simulink model "drone_udp"  (Simulink 8.4)
settings: Solver=ode45  StartTime=0.0  StopTime=300  FixedStep=.01  RelTol=abstol/10  AbsTol=abstol
undefined symbols (not defined in the file or in its folder): A, Cd, g, I, I_motor, m, MaxPropRate, MaxPwmWidth, MinPwmWidth, q0, r0, r1, r2, r3, r4, RateToForce, rho, v0, w0
libraries: instrumentlib x2, simulink x2, dspmtrx3 x2, aerolibutil x1
settings Model: Creator=Mike  LastModifiedBy=Walker
settings SolverCC: ZeroCrossControl=DisableAll
settings DebuggingCC: StrictBusMsg=Warning

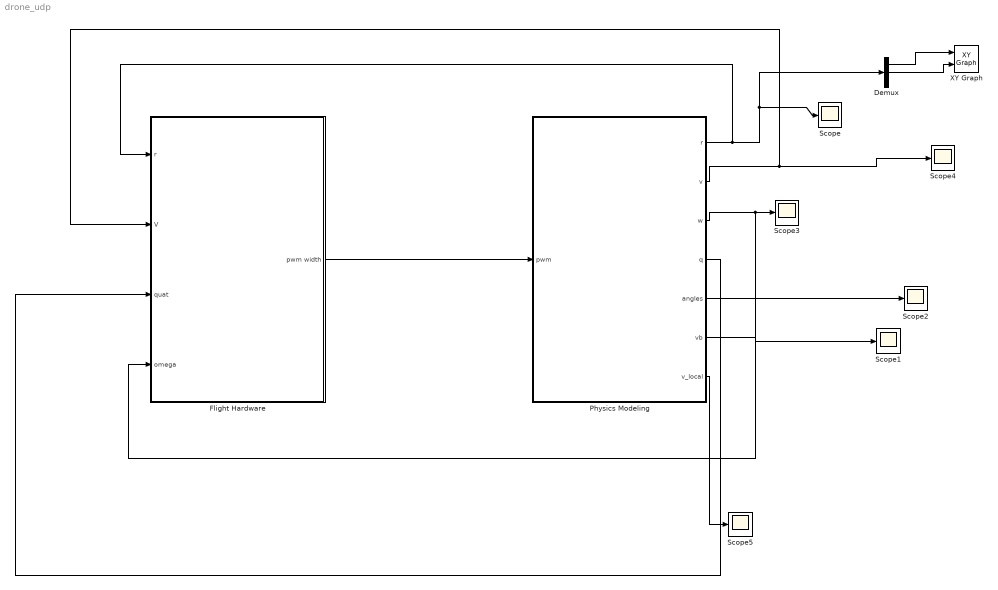
== system drone_udp ==
  Demux : Demux  Outputs=3
  Flight Hardware : Subsystem
  Physics Modeling : Subsystem
  Scope{,1..5} (6 alike) : Scope
      Scope settings: TimeRange=10  YMin=1.25  YMax=5.5
      Scope1 settings: TimeRange=25  YMin=-0.25  YMax=2.75  SaveName=ScopeData7
      Scope2 settings: TimeRange=25  YMin=-0.25  YMax=2.75  SaveName=ScopeData5
      Scope3 settings: TimeRange=50  YMin=-0.0004  YMax=2.5e-005  SaveName=ScopeData13
      Scope4 settings: TimeRange=3.5  YMin=-0.01056459374999874  YMax=0.007040906250001269  SaveName=ScopeData38
      Scope5 settings: TimeRange=25  YMax=65  SaveName=ScopeData10
  XY Graph : simulink/Sinks/XY Graph  xmin=-20  xmax=20  ymin=-20  ymax=20  st=1
  wires:
  Physics Modeling/1(r) -> Scope/1, Demux/1, Flight Hardware/1(r)
  Physics Modeling/5(angles) -> Scope2/1
  Physics Modeling/3(w) -> Scope3/1, Flight Hardware/4(omega)
  Physics Modeling/2(v) -> Scope4/1, Flight Hardware/2(V)
  Physics Modeling/7(v_local) -> Scope5/1
  Physics Modeling/6(vb) -> Scope1/1
  Demux/1 -> XY Graph/1
  Demux/2 -> XY Graph/2
  Flight Hardware/1(pwm width) -> Physics Modeling/1(pwm)
  Physics Modeling/4(q) -> Flight Hardware/3(quat)

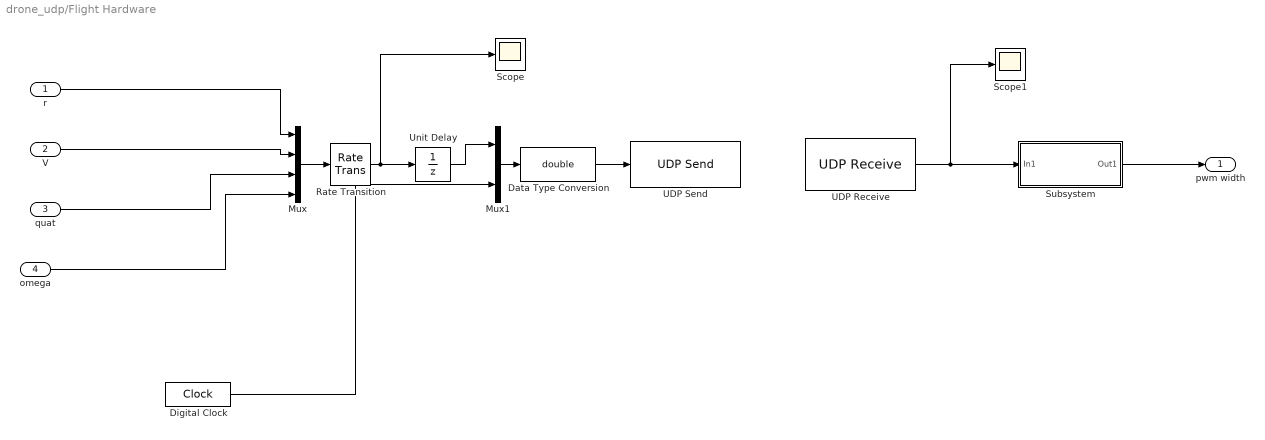
== system drone_udp/Flight Hardware ==
  r : Inport
  V : Inport  Port=2
  quat : Inport  Port=3
  omega : Inport  Port=4
  Data Type Conversion : DataTypeConversion  OutDataTypeStr=double
  Digital Clock : DigitalClock  SampleTime=0.01
  Mux : Mux
  Mux1 : Mux  Inputs=2
  Rate Transition : RateTransition  OutPortSampleTime=0.01
  Scope : Scope
      settings: TimeRange=100
  Scope1 : Scope
      settings: TimeRange=100  YMin=-1e+062  YMax=1e+062  SaveName=ScopeData12
  Subsystem : Subsystem
  UDP Receive : instrumentlib/UDP Receive  Host=127.0.0.1  Port=9091  LocalPort=9091  DataSize=13  EnableBlockingMode=on  Timeout=10  SampleTime=0.01  DataType=double  ByteOrder=LittleEndian
  UDP Send : instrumentlib/UDP Send  Host=127.0.0.1  Port=9090  LocalPort=-1  EnableBlockingMode=off  ByteOrder=LittleEndian
  Unit Delay : UnitDelay  InitialCondition=[r0 v0 q0 w0 ]  SampleTime=-1
  pwm width : Outport
  wires:
  r/1 -> Mux/1
  V/1 -> Mux/2
  omega/1 -> Mux/4
  Data Type Conversion/1 -> UDP Send/1
  quat/1 -> Mux/3
  Mux/1 -> Rate Transition/1
  Rate Transition/1 -> Scope/1, Unit Delay/1
  Subsystem/1(Out1) -> pwm width/1
  UDP Receive/1 -> Scope1/1, Subsystem/1(In1)
  Unit Delay/1 -> Mux1/1
  Digital Clock/1 -> Mux1/2
  Mux1/1 -> Data Type Conversion/1

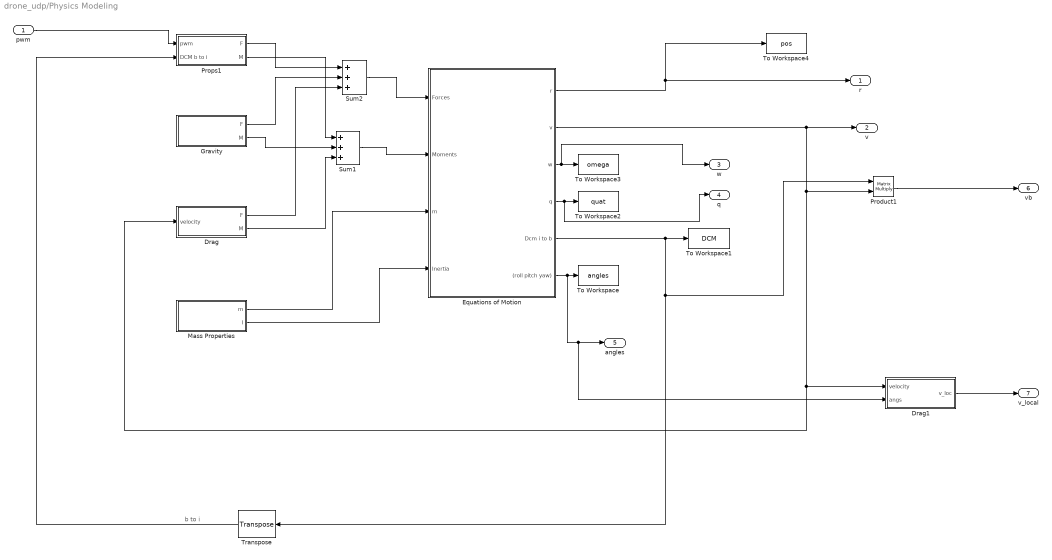
== system drone_udp/Physics Modeling ==
  note: b to i
  pwm : Inport
  Drag : Subsystem
  Drag1 : Subsystem
  Equations of Motion : Subsystem
  Gravity : Subsystem
  Mass Properties : Subsystem
  Product1 : Product  Multiplication=Matrix(*)  RndMeth=Zero
  Props1 : Subsystem
  Sum1 : Sum  Inputs=+++
  Sum2 : Sum  Inputs=+++
  To Workspace : ToWorkspace  VariableName=angles  SampleTime=-1
  To Workspace1 : ToWorkspace  VariableName=DCM  SampleTime=-1
  To Workspace2 : ToWorkspace  VariableName=quat  SampleTime=-1
  To Workspace3 : ToWorkspace  VariableName=omega  SampleTime=-1
  To Workspace4 : ToWorkspace  VariableName=pos  SampleTime=-1
  Transpose : dspmtrx3/Transpose  Hermitian=off  overflowFlag=off
  r : Outport
  v : Outport  Port=2
  w : Outport  Port=3
  q : Outport  Port=4
  angles : Outport  Port=5
  vb : Outport  Port=6
  v_local : Outport  Port=7
  wires:
  Props1/1(F) -> Sum2/1
  Gravity/1(F) -> Sum2/2
  Drag/1(F) -> Sum2/3
  Sum2/1 -> Equations of Motion/1(Forces)
  Props1/2(M) -> Sum1/1
  Gravity/2(M) -> Sum1/2
  Drag/2(M) -> Sum1/3
  Sum1/1 -> Equations of Motion/2(Moments)
  Mass Properties/1(m) -> Equations of Motion/3(m)
  Mass Properties/2(I) -> Equations of Motion/4(Inertia)
  pwm/1 -> Props1/1(pwm)
  Equations of Motion/2(v) -> Drag/1(velocity), Drag1/1(velocity), Product1/2, v/1
  Equations of Motion/1(r) -> To Workspace4/1, r/1
  Equations of Motion/6((roll pitch yaw)) -> To Workspace/1, angles/1, Drag1/2(angs)
  Equations of Motion/5(Dcm i to b) -> To Workspace1/1, Transpose/1, Product1/1
  Equations of Motion/4(q) -> To Workspace2/1, q/1
  Equations of Motion/3(w) -> To Workspace3/1, w/1
  Transpose/1 -> Props1/2("DCM b to i ")
  Product1/1 -> vb/1
  Drag1/1(v_loc) -> v_local/1

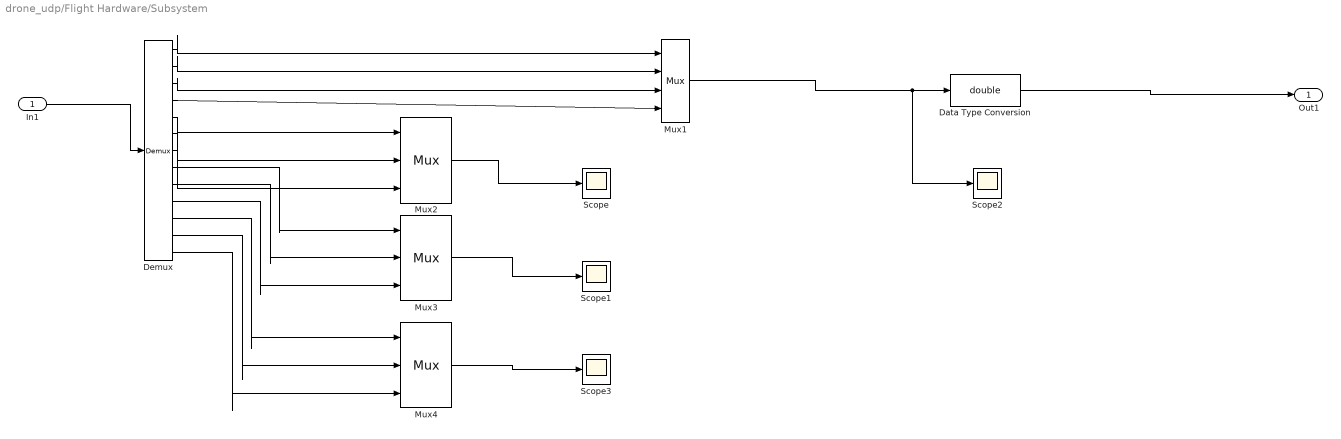
== system drone_udp/Flight Hardware/Subsystem ==
  In1 : Inport
  Data Type Conversion : DataTypeConversion  OutDataTypeStr=double
  Demux : Demux  Outputs=13
  Mux1 : Mux
  Mux2 : Mux  Inputs=3
  Mux3 : Mux  Inputs=3
  Mux4 : Mux  Inputs=3
  Scope{,1..3} (4 alike) : Scope
      Scope settings: YMin=-10  YMax=220  SaveName=ScopeData6
      Scope1 settings: YMin=-1.12743e+008  YMax=-1.02005e+008  SaveName=ScopeData15
      Scope2 settings: TimeRange=3.5  YMin=-2000  YMax=2000  SaveName=ScopeData20
      Scope3 settings: YMin=-0.9  YMax=0.6  SaveName=ScopeData23
  Out1 : Outport
  wires:
  In1/1 -> Demux/1
  Demux/1 -> Mux1/1
  Demux/2 -> Mux1/2
  Demux/3 -> Mux1/3
  Demux/4 -> Mux1/4
  Mux2/1 -> Scope/1
  Demux/5 -> Mux2/1
  Demux/6 -> Mux2/2
  Demux/7 -> Mux2/3
  Data Type Conversion/1 -> Out1/1
  Mux1/1 -> Data Type Conversion/1, Scope2/1
  Demux/8 -> Mux3/1
  Demux/9 -> Mux3/2
  Demux/10 -> Mux3/3
  Mux3/1 -> Scope1/1
  Demux/11 -> Mux4/1
  Demux/12 -> Mux4/2
  Demux/13 -> Mux4/3
  Mux4/1 -> Scope3/1

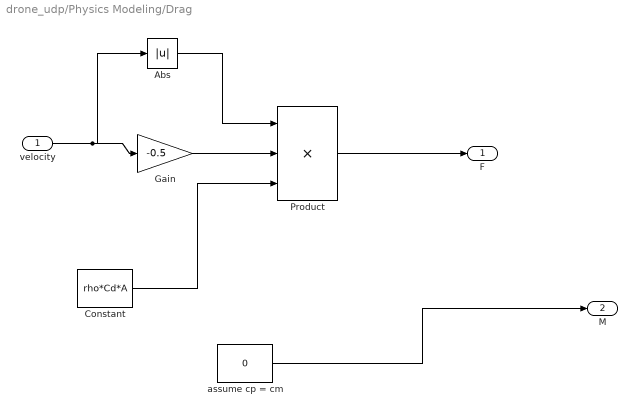
== system drone_udp/Physics Modeling/Drag ==
  velocity : Inport
  Abs : Abs
  Constant : Constant  Value=rho*Cd*A
  Gain : Gain  Gain=-0.5
  Product : Product  Inputs=***  RndMeth=Zero
  assume cp = cm : Constant  Value=0
  F : Outport
  M : Outport  Port=2
  wires:
  velocity/1 -> Abs/1, Gain/1
  Gain/1 -> Product/2
  Abs/1 -> Product/1
  Constant/1 -> Product/3
  assume cp = cm/1 -> M/1
  Product/1 -> F/1

== system drone_udp/Physics Modeling/Drag1 ==
  velocity : Inport
  angs : Inport  Port=2
  Embedded MATLAB Function : MATLAB Function  TreatAsAtomicUnit=on
  Product : Product  Multiplication=Matrix(*)  RndMeth=Zero
  v_loc : Outport
  wires:
  velocity/1 -> Product/2
  Product/1 -> v_loc/1
  angs/1 -> Embedded MATLAB Function/1(u)
  Embedded MATLAB Function/1(y) -> Product/1

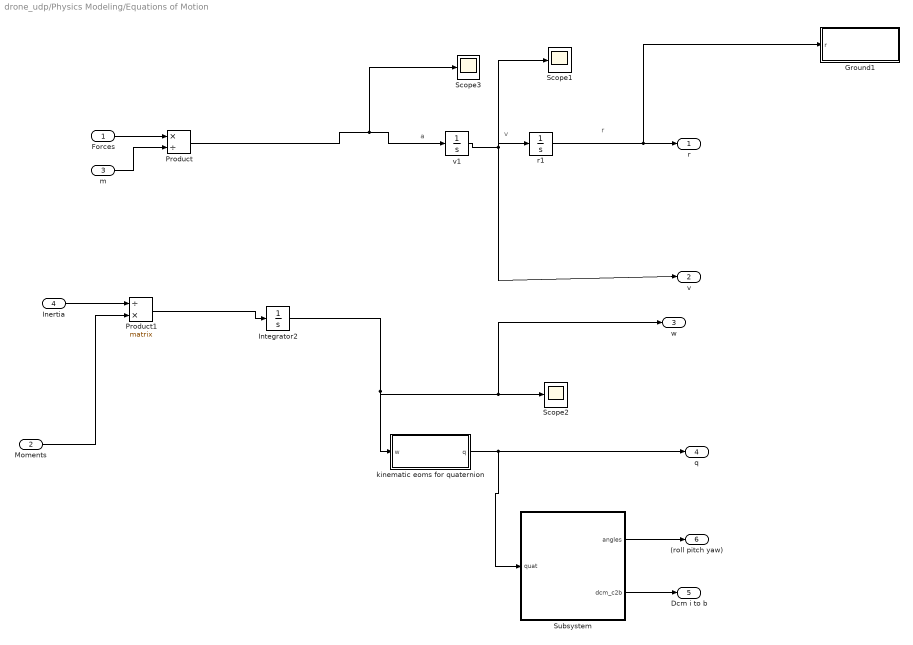
== system drone_udp/Physics Modeling/Equations of Motion ==
  note: a
  note: v
  note: r
  Forces : Inport
  Moments : Inport  Port=2
  m : Inport  Port=3
  Inertia : Inport  Port=4
  Ground1 : Subsystem
  Integrator2 : Integrator  InitialCondition=w0  AbsoluteTolerance=abstol
  Product : Product  Inputs=*/  RndMeth=Zero
  Product1 : Product  Inputs=/*  Multiplication=Matrix(*)  RndMeth=Zero
  Scope1 : Scope
      settings: TimeRange=50  YMin=-2000  YMax=0  SaveName=ScopeData24
  Scope2 : Scope
      settings: TimeRange=50  YMin=-2000  YMax=0  SaveName=ScopeData14
  Scope3 : Scope
      settings: TimeRange=50  YMin=-2000  YMax=0  SaveName=ScopeData25
  Subsystem : Subsystem
  kinematic eoms for quaternion : Subsystem
  r1 : Integrator  InitialCondition=r0  AbsoluteTolerance=abstol
  v1 : Integrator  InitialCondition=v0  AbsoluteTolerance=abstol
  r : Outport
  v : Outport  Port=2
  w : Outport  Port=3
  q : Outport  Port=4
  Dcm i to b : Outport  Port=5
  (roll pitch yaw) : Outport  Port=6
  wires:
  r1/1 -> r/1, Ground1/1(r)
  v1/1 -> r1/1, v/1, Scope1/1
  Forces/1 -> Product/1
  m/1 -> Product/2
  kinematic eoms for quaternion/1(q) -> q/1, Subsystem/1(quat)
  Subsystem/2(dcm_c2b) -> Dcm i to b/1
  Subsystem/1(angles) -> (roll pitch yaw)/1
  Inertia/1 -> Product1/1
  Moments/1 -> Product1/2
  Product/1 -> v1/1, Scope3/1
  Integrator2/1 -> kinematic eoms for quaternion/1(w), Scope2/1, w/1
  Product1/1 -> Integrator2/1

== system drone_udp/Physics Modeling/Gravity ==
  cg=cm in this problem : Constant  Value=0
  mg : Constant  Value=[0;0; -m*g ]
  F : Outport
  M : Outport  Port=2
  wires:
  cg=cm in this problem/1 -> M/1
  mg/1 -> F/1

== system drone_udp/Physics Modeling/Mass Properties ==
  Constant : Constant  Value=m
  a : Constant  Value=I
  m : Outport
  I : Outport  Port=2
  wires:
  a/1 -> I/1
  Constant/1 -> m/1

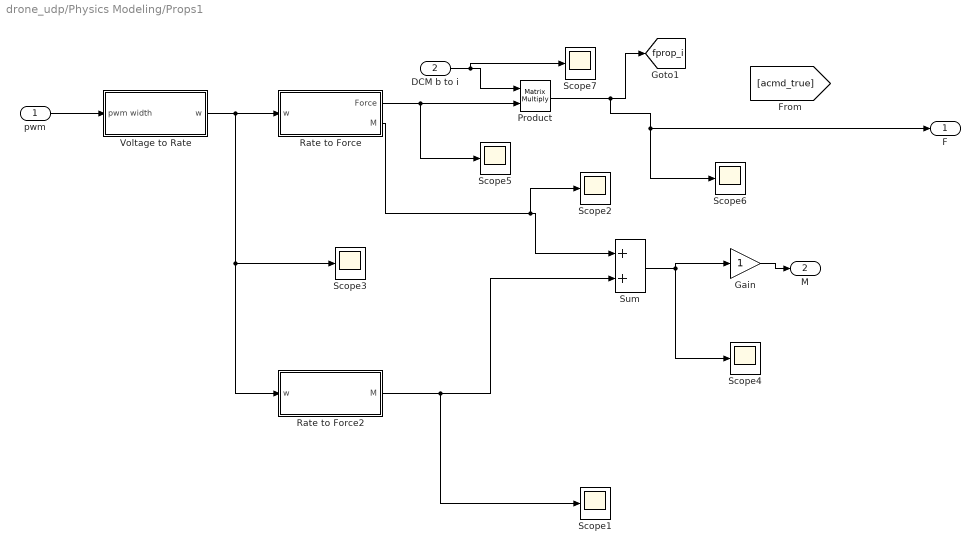
== system drone_udp/Physics Modeling/Props1 ==
  pwm : Inport
  "DCM b to i " : Inport  Port=2
  Gain : Gain
  Product : Product  Multiplication=Matrix(*)  OutDataTypeStr=Inherit: Inherit via back propagation  RndMeth=Nearest
  Rate to Force : Subsystem
  Rate to Force2 : Subsystem
  Scope{1..7} (7 alike) : Scope
      Scope1 settings: TimeRange=50  YMin=0  YMax=200  SaveName=ScopeData2
      Scope2 settings: YMin=-1  YMax=1  SaveName=ScopeData3
      Scope3 settings: TimeRange=50  YMin=2.32987  YMax=2.57513  SaveName=ScopeData4
      Scope4 settings: TimeRange=6.110074626865668  YMin=-3.63961038961039e-009  YMax=-3.405844155844153e-009  SaveName=ScopeData11
      Scope5 settings: TimeRange=50  YMin=0  YMax=40  SaveName=ScopeData9
      Scope6 settings: TimeRange=50  YMin=0  YMax=40  SaveName=ScopeData59
      Scope7 settings: TimeRange=0.2158273381295004  YMin=-0.1758241758241754  YMax=0.1318681318681321  SaveName=ScopeData62
  Sum : Sum
  Voltage to Rate : Subsystem
  F : Outport
  M : Outport  Port=2
  tag scope: fprop_i=global
  wires:
  pwm/1 -> Voltage to Rate/1(pwm width)
  Voltage to Rate/1(w) -> Rate to Force/1(w), Rate to Force2/1(w), Scope3/1
  Sum/1 -> Scope4/1, Gain/1
  Rate to Force/2(M) -> Sum/1, Scope2/1
  Rate to Force2/1(M) -> Sum/2, Scope1/1
  Product/1 -> [fprop_i], Scope6/1, F/1
  "DCM b to i "/1 -> Product/1, Scope7/1
  Rate to Force/1(Force) -> Product/2, Scope5/1
  Gain/1 -> M/1

== system drone_udp/Physics Modeling/Equations of Motion/Ground1 ==
  r : Inport
  Compare To Zero : simulink/Logic and Bit Operations/Compare To Zero  SystemSampleTime=-1  relop=<=  LogicOutDataTypeMode=boolean  ZeroCross=off
  Demux : Demux  Outputs=3
  Stop Simulation : Stop
  Terminator : Terminator
  Terminator1 : Terminator
  wires:
  r/1 -> Demux/1
  Demux/1 -> Terminator/1
  Demux/2 -> Terminator1/1
  Demux/3 -> Compare To Zero/1
  Compare To Zero/1 -> Stop Simulation/1

== system drone_udp/Physics Modeling/Equations of Motion/Subsystem ==
  note: Based on Prof Howell AAE 440 Notes
  note: C is row notation so transpose it!
  quat : Inport
  Transpose1 : dspmtrx3/Transpose  SystemSampleTime=-1  Hermitian=off  overflowFlag=off
  solve direction cosine matrix : Subsystem
  angles : Outport
  dcm_c2b : Outport  Port=2
  wires:
  quat/1 -> solve direction cosine matrix/1(quat)
  solve direction cosine matrix/2(roll pitch yaw) -> angles/1
  solve direction cosine matrix/1(C) -> Transpose1/1
  Transpose1/1 -> dcm_c2b/1

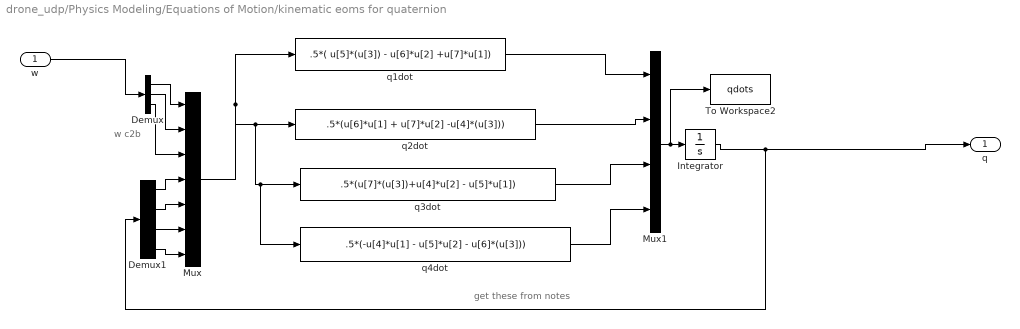
== system drone_udp/Physics Modeling/Equations of Motion/kinematic eoms for quaternion ==
  note: get these from notes
  note: w c2b
  w : Inport
  Demux : Demux  Outputs=3
  Demux1 : Demux
  Integrator : Integrator  InitialCondition=q0  IgnoreLimit=on
  Mux : Mux  Inputs=7
  Mux1 : Mux
  To Workspace2 : ToWorkspace  VariableName=qdots  SampleTime=-1
  q1dot : Fcn  Expr=.5*( u[5]*(u[3]) - u[6]*u[2] +u[7]*u[1])
  q2dot : Fcn  Expr=.5*(u[6]*u[1] + u[7]*u[2] -u[4]*(u[3]))
  q3dot : Fcn  Expr=.5*(u[7]*(u[3])+u[4]*u[2] - u[5]*u[1])
  q4dot : Fcn  Expr=.5*(-u[4]*u[1] - u[5]*u[2] - u[6]*(u[3]))
  q : Outport
  wires:
  Mux1/1 -> Integrator/1, To Workspace2/1
  Integrator/1 -> Demux1/1, q/1
  q4dot/1 -> Mux1/4
  q3dot/1 -> Mux1/3
  q2dot/1 -> Mux1/2
  q1dot/1 -> Mux1/1
  Mux/1 -> q1dot/1, q2dot/1, q3dot/1, q4dot/1
  w/1 -> Demux/1
  Demux/1 -> Mux/1
  Demux/2 -> Mux/2
  Demux/3 -> Mux/3
  Demux1/1 -> Mux/4
  Demux1/2 -> Mux/5
  Demux1/3 -> Mux/6
  Demux1/4 -> Mux/7

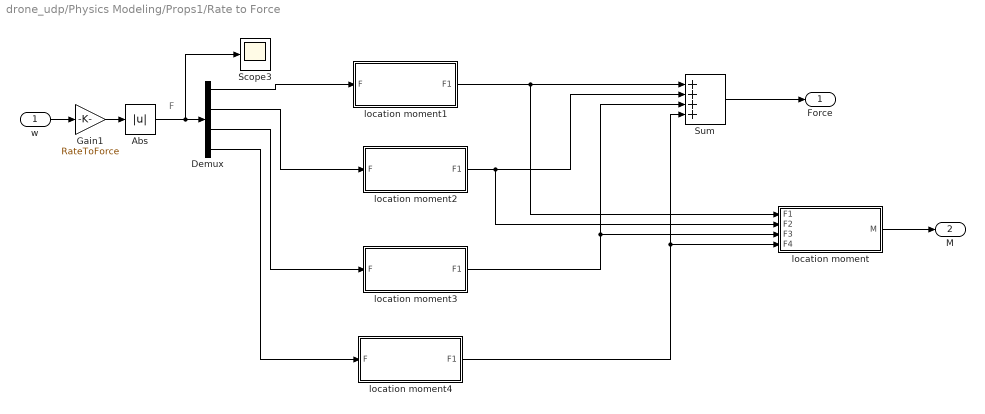
== system drone_udp/Physics Modeling/Props1/Rate to Force ==
  note: F
  w : Inport
  Abs : Abs
  Demux : Demux
  Gain1 : Gain  Gain=RateToForce
  Scope3 : Scope
      settings: TimeRange=50  YMin=2.32987  YMax=2.57513  SaveName=ScopeData8
  Sum : Sum  Inputs=++++
  location moment : Subsystem
  location moment1 : Subsystem
  location moment2 : Subsystem
  location moment3 : Subsystem
  location moment4 : Subsystem
  Force : Outport
  M : Outport  Port=2
  wires:
  location moment/1(M) -> M/1
  Sum/1 -> Force/1
  location moment1/1(F1) -> Sum/1, location moment/1(F1)
  location moment2/1(F1) -> Sum/2, location moment/2(F2)
  location moment3/1(F1) -> Sum/3, location moment/3(F3)
  location moment4/1(F1) -> Sum/4, location moment/4(F4)
  Demux/1 -> location moment1/1(F)
  Demux/2 -> location moment2/1(F)
  Demux/3 -> location moment3/1(F)
  Demux/4 -> location moment4/1(F)
  Abs/1 -> Demux/1, Scope3/1
  w/1 -> Gain1/1
  Gain1/1 -> Abs/1

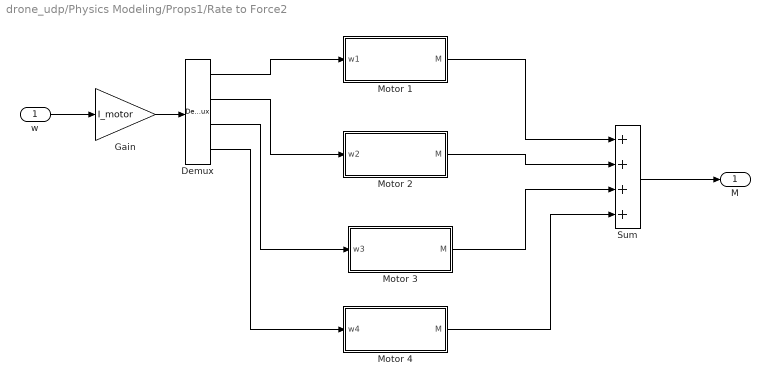
== system drone_udp/Physics Modeling/Props1/Rate to Force2 ==
  w : Inport
  Demux : Demux
  Gain : Gain  Gain=I_motor
  Motor 1 : Subsystem
  Motor 2 : Subsystem
  Motor 3 : Subsystem
  Motor 4 : Subsystem
  Sum : Sum  Inputs=++++
  M : Outport
  wires:
  w/1 -> Gain/1
  Gain/1 -> Demux/1
  Demux/1 -> Motor 1/1(w1)
  Demux/2 -> Motor 2/1(w2)
  Demux/4 -> Motor 4/1(w4)
  Motor 3/1(M) -> Sum/3
  Motor 4/1(M) -> Sum/4
  Motor 2/1(M) -> Sum/2
  Motor 1/1(M) -> Sum/1
  Sum/1 -> M/1
  Demux/3 -> Motor 3/1(w3)

== system drone_udp/Physics Modeling/Props1/Voltage to Rate ==
  pwm width : Inport
  Constant : Constant  Value=MinPwmWidth
  Gain : Gain  Gain=1/(MaxPwmWidth - MinPwmWidth)
  Gain1 : Gain  Gain=MaxPropRate
  Rotation Direction : Gain  Gain=[1 -1 1 -1]
  Sum : Sum  Inputs=|+-
  w : Outport
  wires:
  Constant/1 -> Sum/2
  Sum/1 -> Gain/1
  Rotation Direction/1 -> w/1
  pwm width/1 -> Sum/1
  Gain1/1 -> Rotation Direction/1
  Gain/1 -> Gain1/1

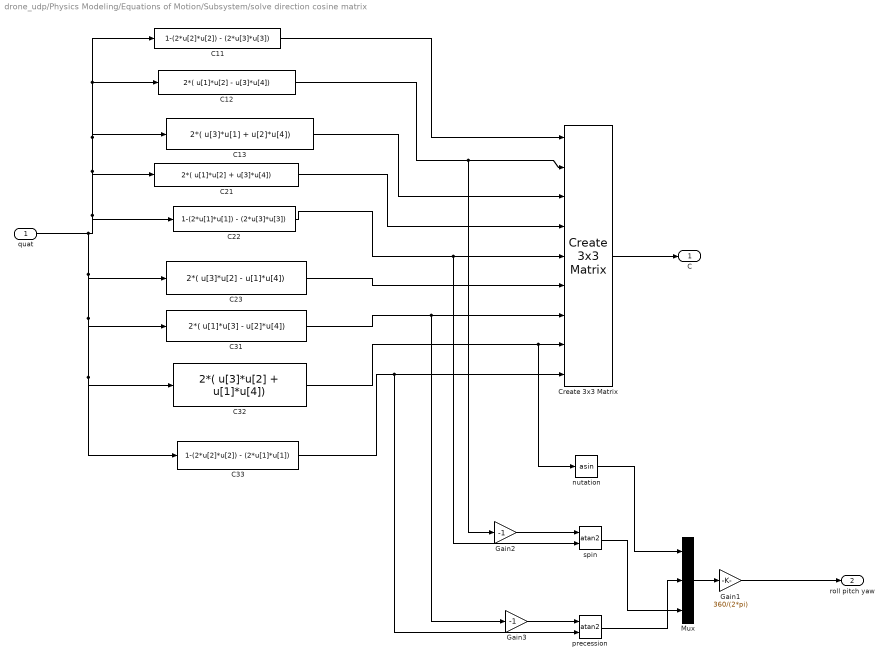
== system drone_udp/Physics Modeling/Equations of Motion/Subsystem/solve direction cosine matrix ==
  quat : Inport
  C11 : Fcn  Expr=1-(2*u[2]*u[2]) - (2*u[3]*u[3])
  C12 : Fcn  Expr=2*( u[1]*u[2] - u[3]*u[4])
  C13 : Fcn  Expr=2*( u[3]*u[1] + u[2]*u[4])
  C21 : Fcn  Expr=2*( u[1]*u[2] + u[3]*u[4])
  C22 : Fcn  Expr=1-(2*u[1]*u[1]) - (2*u[3]*u[3])
  C23 : Fcn  Expr=2*( u[3]*u[2] - u[1]*u[4])
  C31 : Fcn  Expr=2*( u[1]*u[3] - u[2]*u[4])
  C32 : Fcn  Expr=2*( u[3]*u[2] + u[1]*u[4])
  C33 : Fcn  Expr=1-(2*u[2]*u[2]) - (2*u[1]*u[1])
  Create 3x3 Matrix : aerolibutil/Create 3x3 Matrix  SystemSampleTime=-1
  Gain1 : Gain  Gain=360/(2*pi)
  Gain2 : Gain  Gain=-1
  Gain3 : Gain  Gain=-1
  Mux : Mux  Inputs=3
  nutation : Trigonometry  Operator=asin
  precession : Trigonometry  Operator=atan2
  spin : Trigonometry  Operator=atan2
  C : Outport
  roll pitch yaw : Outport  Port=2
  wires:
  Create 3x3 Matrix/1 -> C/1
  quat/1 -> C22/1, C13/1, C11/1, C12/1, C21/1, C23/1, C31/1, C33/1, C32/1
  C11/1 -> Create 3x3 Matrix/1
  C12/1 -> Create 3x3 Matrix/2, Gain2/1
  C13/1 -> Create 3x3 Matrix/3
  C21/1 -> Create 3x3 Matrix/4
  C22/1 -> Create 3x3 Matrix/5, spin/2
  C23/1 -> Create 3x3 Matrix/6
  C31/1 -> Create 3x3 Matrix/7, Gain3/1
  C32/1 -> Create 3x3 Matrix/8, nutation/1
  C33/1 -> Create 3x3 Matrix/9, precession/2
  Gain1/1 -> roll pitch yaw/1
  Mux/1 -> Gain1/1
  Gain2/1 -> spin/1
  Gain3/1 -> precession/1
  nutation/1 -> Mux/1
  spin/1 -> Mux/3
  precession/1 -> Mux/2

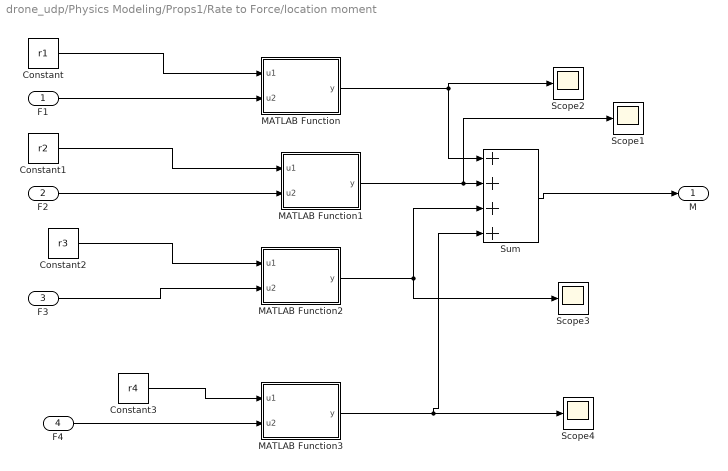
== system drone_udp/Physics Modeling/Props1/Rate to Force/location moment ==
  F1 : Inport
  F2 : Inport  Port=2
  F3 : Inport  Port=3
  F4 : Inport  Port=4
  Constant : Constant  Value=r1
  Constant1 : Constant  Value=r2
  Constant2 : Constant  Value=r3
  Constant3 : Constant  Value=r4
  MATLAB Function : MATLAB Function  TreatAsAtomicUnit=on
  MATLAB Function1 : MATLAB Function  TreatAsAtomicUnit=on
  MATLAB Function2 : MATLAB Function  TreatAsAtomicUnit=on
  MATLAB Function3 : MATLAB Function  TreatAsAtomicUnit=on
  Scope{1..4} (4 alike) : Scope
      Scope1 settings: YMin=-1  YMax=1  SaveName=ScopeData17
      Scope2 settings: TimeRange=50  YMin=-1  YMax=1  SaveName=ScopeData16
      Scope3 settings: TimeRange=50  YMin=-1  YMax=1  SaveName=ScopeData18
      Scope4 settings: TimeRange=50  YMin=-1  YMax=1  SaveName=ScopeData19
  Sum : Sum  Inputs=++++
  M : Outport
  wires:
  F2/1 -> MATLAB Function1/2(u2)
  F1/1 -> MATLAB Function/2(u2)
  Constant/1 -> MATLAB Function/1(u1)
  Sum/1 -> M/1
  MATLAB Function/1(y) -> Scope2/1, Sum/1
  MATLAB Function1/1(y) -> Sum/2, Scope1/1
  MATLAB Function2/1(y) -> Scope3/1, Sum/3
  MATLAB Function3/1(y) -> Sum/4, Scope4/1
  Constant1/1 -> MATLAB Function1/1(u1)
  Constant2/1 -> MATLAB Function2/1(u1)
  F3/1 -> MATLAB Function2/2(u2)
  F4/1 -> MATLAB Function3/2(u2)
  Constant3/1 -> MATLAB Function3/1(u1)

== system drone_udp/Physics Modeling/Props1/Rate to Force/location moment1 ==
  F : Inport
  Constant : Constant  Value=0
  Mux : Mux  Inputs=3
  F1 : Outport
  wires:
  Constant/1 -> Mux/2, Mux/1
  F/1 -> Mux/3
  Mux/1 -> F1/1

== system drone_udp/Physics Modeling/Props1/Rate to Force/location moment2 ==
  F : Inport
  Constant : Constant  Value=0
  Mux : Mux  Inputs=3
  F1 : Outport
  wires:
  Constant/1 -> Mux/2, Mux/1
  F/1 -> Mux/3
  Mux/1 -> F1/1

== system drone_udp/Physics Modeling/Props1/Rate to Force/location moment3 ==
  F : Inport
  Constant : Constant  Value=0
  Mux : Mux  Inputs=3
  F1 : Outport
  wires:
  Constant/1 -> Mux/2, Mux/1
  F/1 -> Mux/3
  Mux/1 -> F1/1

== system drone_udp/Physics Modeling/Props1/Rate to Force/location moment4 ==
  F : Inport
  Constant : Constant  Value=0
  Mux : Mux  Inputs=3
  F1 : Outport
  wires:
  Constant/1 -> Mux/2, Mux/1
  F/1 -> Mux/3
  Mux/1 -> F1/1

== system drone_udp/Physics Modeling/Props1/Rate to Force2/Motor 1 ==
  w1 : Inport
  Constant : Constant  Value=0
  Gain : Gain
  Mux : Mux  Inputs=3
  M : Outport
  wires:
  Mux/1 -> M/1
  Constant/1 -> Mux/2, Mux/1
  Gain/1 -> Mux/3
  w1/1 -> Gain/1

== system drone_udp/Physics Modeling/Props1/Rate to Force2/Motor 2 ==
  w2 : Inport
  Constant : Constant  Value=0
  Gain : Gain
  Mux : Mux  Inputs=3
  M : Outport
  wires:
  Mux/1 -> M/1
  Constant/1 -> Mux/2, Mux/1
  Gain/1 -> Mux/3
  w2/1 -> Gain/1

== system drone_udp/Physics Modeling/Props1/Rate to Force2/Motor 3 ==
  w3 : Inport
  Constant : Constant  Value=0
  Gain : Gain
  Mux : Mux  Inputs=3
  M : Outport
  wires:
  Mux/1 -> M/1
  Constant/1 -> Mux/2, Mux/1
  Gain/1 -> Mux/3
  w3/1 -> Gain/1

== system drone_udp/Physics Modeling/Props1/Rate to Force2/Motor 4 ==
  w4 : Inport
  Constant : Constant  Value=0
  Gain : Gain
  Mux : Mux  Inputs=3
  M : Outport
  wires:
  Mux/1 -> M/1
  Constant/1 -> Mux/2, Mux/1
  Gain/1 -> Mux/3
  w4/1 -> Gain/1

== matlab function Physics Modeling/Drag1/Embedded MATLAB Function ==
  data: u input double; y output double
function y = fcn(u)
%#eml

y = [ cosd(u(3)), sind(u(3)) , 0;  -sind(u(3)), cosd(u(3)) 0 ; 0 , 0 , 1];

== matlab function Physics Modeling/Props1/Rate to Force/location moment/MATLAB Function ==
  data: u1 input double; y output double; u2 input double
function y = fcn(u1,u2)
%#codegen

y = cross(u1,u2);

== matlab function Physics Modeling/Props1/Rate to Force/location moment/MATLAB Function1 ==
  data: u1 input double; y output double; u2 input double
function y = fcn(u1,u2)
%#codegen

y = cross(u1,u2);

== matlab function Physics Modeling/Props1/Rate to Force/location moment/MATLAB Function2 ==
  data: u1 input double; y output double; u2 input double
function y = fcn(u1,u2)
%#codegen

y = cross(u1,u2);

== matlab function Physics Modeling/Props1/Rate to Force/location moment/MATLAB Function3 ==
  data: u1 input double; y output double; u2 input double
function y = fcn(u1,u2)
%#codegen

y = cross(u1,u2);
